simulink model "FOC_PIL_StateMachine_Sim"  (R2022b)
settings: Solver=FixedStepAuto  StartTime=0.0  StopTime=2.5  FixedStep=Ts_PIL  RelTol=1e-3
values from neighbouring files (symbols this model uses):
  Tctr = Ts    (= 5e-05)    [FOC_Config.m]
undefined symbols (not defined in the file or in its folder): motor
libraries: mcbplantlib x1, autolibpmsminterior x1
settings Model: Creator=k  LastModifiedBy=Administrator
settings SolverCC: AlgebraicLoopSolver=TrustRegion
settings DebuggingCC: UnconnectedInputMsg=warning  UnconnectedOutputMsg=warning  UnconnectedLineMsg=warning  SFMachineParentedDataDiag=warning
settings ModelReferenceCC: EnableRefExpFcnMdlSchedulingChecks=on
settings RTWCC: DLArmComputeVersion=19.05

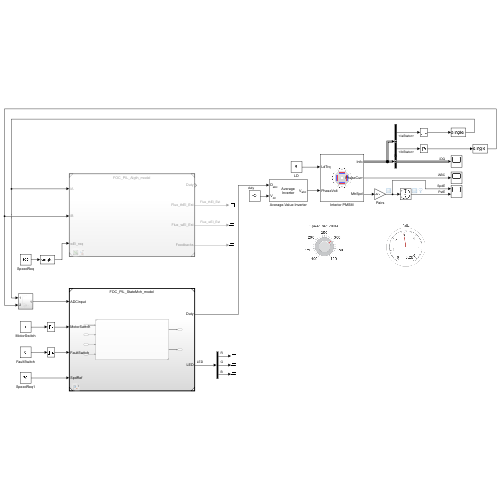
[thumbnail: Simulink's stored preview of the top-level diagram]
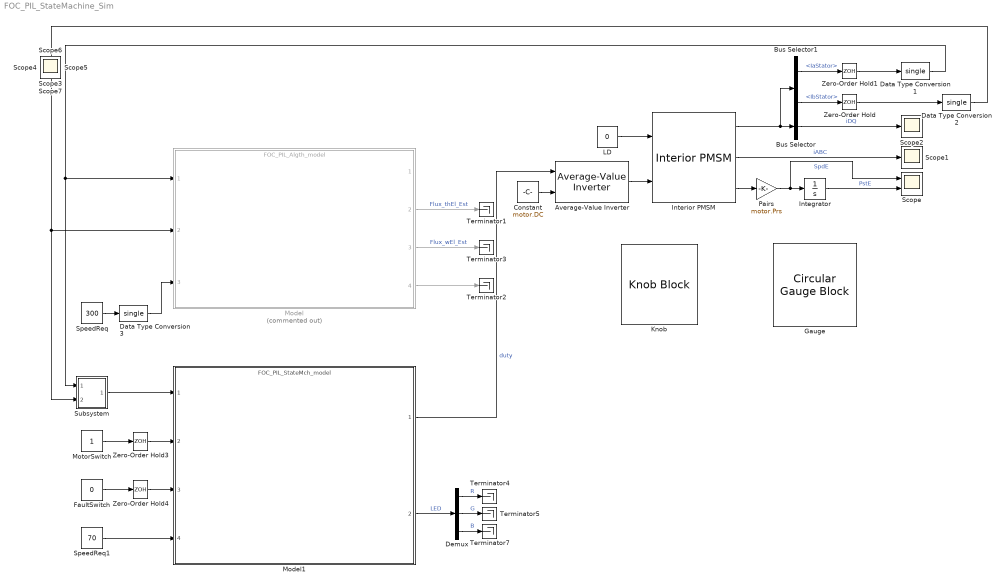
== system FOC_PIL_StateMachine_Sim ==
  Average-Value Inverter : mcbplantlib/Average-Value Inverter
  Bus Selector : BusSelector  OutputSignals=IdSync,IqSync  OutputAsBus=on
  Bus Selector1 : BusSelector  OutputSignals=IaStator,IbStator
  Constant : Constant  Value=motor.DC
  Data Type Conversion1 : DataTypeConversion  OutDataTypeStr=single  SaturateOnIntegerOverflow=off  RndMeth=Floor
  Data Type Conversion2 : DataTypeConversion  OutDataTypeStr=single  SaturateOnIntegerOverflow=off  RndMeth=Floor
  Data Type Conversion3 : DataTypeConversion  OutDataTypeStr=single  SaturateOnIntegerOverflow=off  RndMeth=Floor
  Demux : Demux  Outputs=3
  FaultSwitch : Constant  Value=0  OutDataTypeStr=boolean
  Gauge : CircularGaugeBlock  ScaleMax=6.28  TickInterval=1
  Integrator : Integrator  WrapState=on  WrappedStateUpperValue=2*pi  WrappedStateLowerValue=0
  Interior PMSM : autolibpmsminterior/Interior PMSM  port_config=Torque  sim_type=Continuous  Ts=0.001  P=motor.Prs  Rs=motor.Rs  Ldq=[motor.Ld motor.Lq]  KConstText=Permanent flux linkage constant (lambda_pm):  lambda_pm=motor.Flux  Ke=159.9771  mechanical=[motor.J, motor.B, motor.Tf]  idq0=[0 0]  theta_init=0  omega_init=0  KConst=motor.Flux  lambda_pm_calc=motor.Flux  Kt=0.07  RefBlkName='autolibpmsminterior/Interior PMSM'  aMode=5
  Knob : KnobBlock  ScaleMin=100  ScaleMax=400
  LD : Constant  Value=0
  Model : ModelReference  Commented=on  ModelNameDialog=FOC_PIL_Algth_model.slx  SimulationMode=Normal  ModelReferenceVersion=5.2
  Model1 : ModelReference  ModelNameDialog=FOC_PIL_StateMch_model.slx  SimulationMode=Normal  ModelReferenceVersion=5.25
  MotorSwitch : Constant  OutDataTypeStr=boolean
  Pairs : Gain  Gain=motor.Prs
  Scope : Scope  NumInputPorts=2
  Scope{1..7} (7 alike) : Scope
  SpeedReq : Constant  Value=300
  SpeedReq1 : Constant  Value=70  OutDataTypeStr=int16
  Subsystem : Subsystem
  Terminator{1..5,7} (6 alike) : Terminator
  Zero-Order Hold{,1,3..4} (4 alike) : ZeroOrderHold  SampleTime=Tctr
  wires:
  Bus Selector/1 -> Scope2/1  "iDQ"
  LD/1 -> Interior PMSM/1
  Interior PMSM/1 -> Bus Selector1/1, Bus Selector/1
  Bus Selector1/1 -> Zero-Order Hold1/1  "<IaStator>"
  Pairs/1 -> Integrator/1, Scope/1  "SpdE"
  Interior PMSM/2 -> Scope1/1  "iABC"
  Bus Selector1/2 -> Zero-Order Hold/1  "<IbStator>"
  Interior PMSM/3 -> Pairs/1
  Model1/1 -> Average-Value Inverter/1  "duty"
  Average-Value Inverter/1 -> Interior PMSM/2
  Constant/1 -> Average-Value Inverter/2
  Data Type Conversion1/1 -> Model/1, Subsystem/1(In1)
  Data Type Conversion2/1 -> Subsystem/2(In2), Model/2
  Data Type Conversion3/1 -> Model/3
  SpeedReq/1 -> Data Type Conversion3/1
  Model/2 -> Terminator1/1  "Flux_thEl_Est"
  Model/3 -> Terminator3/1  "Flux_wEl_Est"
  Model/4 -> Terminator2/1
  Integrator/1 -> Scope/2  "PstE"
  Zero-Order Hold/1 -> Data Type Conversion2/1
  Zero-Order Hold1/1 -> Data Type Conversion1/1
  MotorSwitch/1 -> Zero-Order Hold3/1
  Model1/2 -> Demux/1  "LED"
  Zero-Order Hold3/1 -> Model1/2
  FaultSwitch/1 -> Zero-Order Hold4/1
  Demux/1 -> Terminator4/1  "R"
  Zero-Order Hold4/1 -> Model1/3
  Demux/3 -> Terminator7/1  "B"
  Demux/2 -> Terminator5/1  "G"
  Subsystem/1(Out1) -> Model1/1
  SpeedReq1/1 -> Model1/4

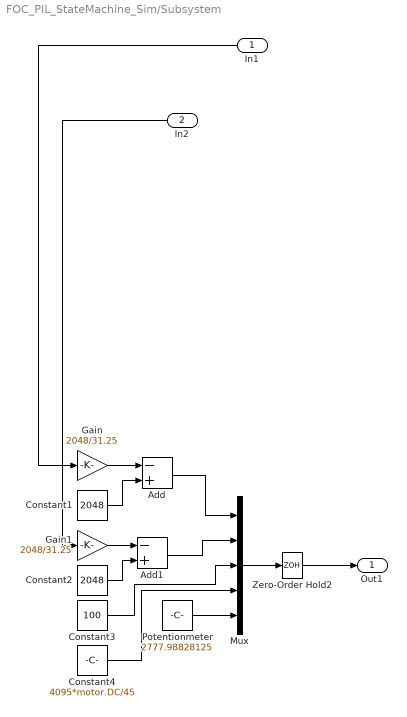
== system FOC_PIL_StateMachine_Sim/Subsystem ==
  In1 : Inport
  In2 : Inport  Port=2
  Add : Sum  Inputs=-+  AccumDataTypeStr=uint16
  Add1 : Sum  Inputs=-+  AccumDataTypeStr=uint16
  Constant1 : Constant  Value=2048  OutDataTypeStr=uint16
  Constant2 : Constant  Value=2048  OutDataTypeStr=uint16
  Constant3 : Constant  Value=100  OutDataTypeStr=uint16
  Constant4 : Constant  Value=4095*motor.DC/45  OutDataTypeStr=uint16
  Gain : Gain  Gain=2048/31.25  OutDataTypeStr=uint16
  Gain1 : Gain  Gain=2048/31.25  OutDataTypeStr=uint16
  Mux : Mux  Inputs=5
  Potentionmeter : Constant  Value=2777.98828125  OutDataTypeStr=uint16
  Zero-Order Hold2 : ZeroOrderHold  SampleTime=Tctr
  Out1 : Outport
  wires:
  Gain1/1 -> Add1/1
  Add/1 -> Mux/1
  Constant1/1 -> Add/2
  Mux/1 -> Zero-Order Hold2/1
  Constant4/1 -> Mux/4
  Zero-Order Hold2/1 -> Out1/1
  Potentionmeter/1 -> Mux/5
  Constant2/1 -> Add1/2
  Constant3/1 -> Mux/3
  Gain/1 -> Add/1
  Add1/1 -> Mux/2
  In1/1 -> Gain/1
  In2/1 -> Gain1/1
